simulink model "verify_HeatExchanger_mdl_2019a"  (R2019a)
settings: Solver=ode45  StartTime=0.0  StopTime=5930  MaxStep=1  RelTol=1e-3  EnableMultiTasking=on
libraries: carnot x9
settings Model: Creator=drhf  LastModifiedBy=P41573
settings DataIOCC: SaveFormat=Array  SignalLoggingSaveFormat=ModelDataLogs  SignalLogging=off  DSMLogging=off  ReturnWorkspaceOutputs=off
settings OptimizationCC: ExpressionDepthLimit=2147483647  LifeSpan=inf
settings DebuggingCC: UnderspecifiedInitializationDetection=Classic  MergeDetectMultiDrivingBlocksExec=none  SolverPrmCheckMsg=warning  FcnCallInpInsideContextMsg=warning  StateNameClashWarn=warning  SFUnexpectedBacktrackingDiag=warning  SFNoUnconditionalDefaultTransitionDiag=warning  SFExecutionAtInitializationDiag=none  ArithmeticOperatorsInVariantConditions=warning
settings HardwareCC: ProdBitPerPointer=32  ProdBitPerSizeT=32  ProdBitPerPtrDiffT=32  ProdLargestAtomicFloat=None  ProdIntDivRoundTo=Undefined  ProdEndianess=Unspecified  ProdWordSize=32  ProdHWDeviceType=32-bit Generic
settings ModelReferenceCC: PropagateSignalLabelsOutOfModel=off
settings SFSimCC: SimUseLocalCustomCode=off
settings RTWCC: RTWUseLocalCustomCode=off
settings CodeAppCC: StateflowObjectComments=on
settings GRTTargetCC: TargetLangStandard=C89/C90 (ANSI)  GeneratePreprocessorConditionals=Disable all  CombineOutputUpdateFcns=off  GRTInterface=on
settings ConfigComp: CovMetricSettings=dw  CovHtmlReporting=on  CovSaveCumulativeToWorkspaceVar=on  CovSaveSingleToWorkspaceVar=on  CovExternalEMLEnable=off

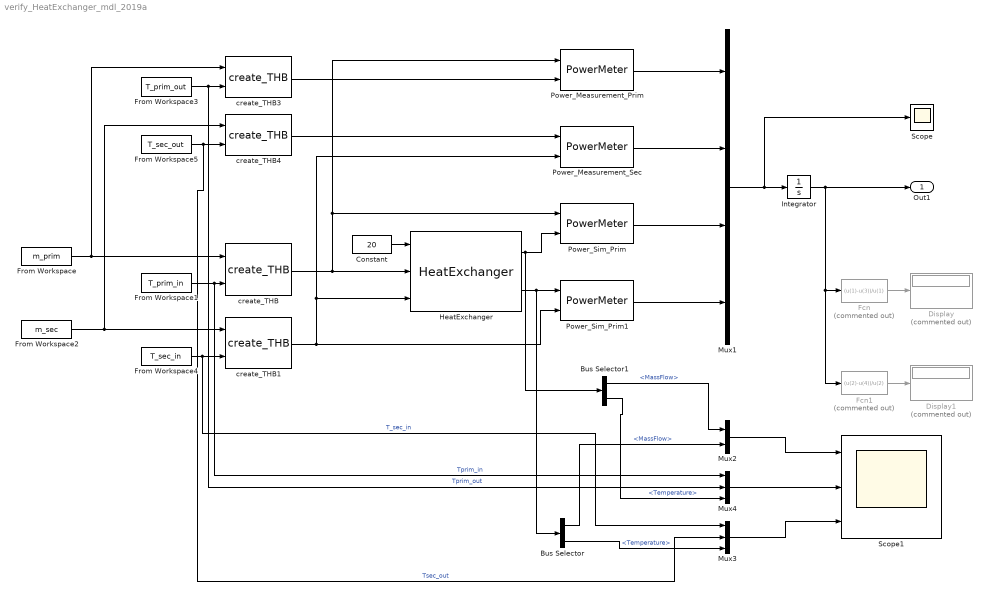
== system verify_HeatExchanger_mdl_2019a ==
  Bus Selector : BusSelector  OutputSignals=MassFlow,Temperature
  Bus Selector1 : BusSelector  OutputSignals=MassFlow,Temperature
  Constant : Constant  Value=20
  Display : Display  Commented=on
  Display1 : Display  Commented=on
  Fcn : Fcn  Commented=on  Expr=(u(1)-u(3))/u(1)
  Fcn1 : Fcn  Commented=on  Expr=(u(2)-u(4))/u(2)
  From Workspace : FromWorkspace  VariableName=m_prim  SampleTime=0
  From Workspace1 : FromWorkspace  VariableName=T_prim_in  SampleTime=0
  From Workspace2 : FromWorkspace  VariableName=m_sec  SampleTime=0
  From Workspace3 : FromWorkspace  VariableName=T_prim_out  SampleTime=0
  From Workspace4 : FromWorkspace  VariableName=T_sec_in  SampleTime=0
  From Workspace5 : FromWorkspace  VariableName=T_sec_out  SampleTime=0
  HeatExchanger : carnot/Source/Heat_Exchanger/HeatExchanger  flowtype=1  ua0=2100  uahot=[0.07 0.41]  uacold=[0.1 0.7]  ualoss=1  cap=8000  linh=20  quah=10  linc=20  quac=10  t0=20
      settings: SourceProductName=Carnot
  Integrator : Integrator
  Mux1 : Mux
  Mux2 : Mux  Inputs=2
  Mux3 : Mux  Inputs=3
  Mux4 : Mux  Inputs=3
  Power_Measurement_Prim : carnot/Control/PowerMeter
      settings: SourceProductName=Carnot
  Power_Measurement_Sec : carnot/Control/PowerMeter
      settings: SourceProductName=Carnot
  Power_Sim_Prim : carnot/Control/PowerMeter
      settings: SourceProductName=Carnot
  Power_Sim_Prim1 : carnot/Control/PowerMeter
      settings: SourceProductName=Carnot
  Scope : Scope
  Scope1 : Scope  NumInputPorts=3
  create_THB{,1,3..4} (4 alike) : carnot/Source/Simple/create_THB  p=1e5  fluid=Water  mix=0  mix2=0  mix3=0  dia=0  hgt=0  mID=No Pressure Drop
      settings: SourceProductName=Carnot
  Out1 : Outport
  wires:
  create_THB/1 -> HeatExchanger/2, Power_Sim_Prim/1, Power_Measurement_Prim/1
  create_THB1/1 -> Power_Measurement_Sec/2, HeatExchanger/3, Power_Sim_Prim1/2
  Constant/1 -> HeatExchanger/1
  From Workspace/1 -> create_THB3/1, create_THB/1
  From Workspace2/1 -> create_THB4/1, create_THB1/1
  From Workspace1/1 -> Mux4/1, create_THB/2  "Tprim_in"
  From Workspace3/1 -> Mux4/2, create_THB3/2  "Tprim_out"
  create_THB3/1 -> Power_Measurement_Prim/2
  Power_Measurement_Prim/1 -> Mux1/1
  Power_Sim_Prim/1 -> Mux1/3
  Power_Measurement_Sec/1 -> Mux1/2
  HeatExchanger/1 -> Bus Selector1/1, Power_Sim_Prim/2
  HeatExchanger/2 -> Bus Selector/1, Power_Sim_Prim1/1
  From Workspace4/1 -> Mux3/1, create_THB1/2  "T_sec_in"
  From Workspace5/1 -> Mux3/2, create_THB4/2  "Tsec_out"
  create_THB4/1 -> Power_Measurement_Sec/1
  Power_Sim_Prim1/1 -> Mux1/4
  Mux1/1 -> Integrator/1, Scope/1
  Integrator/1 -> Out1/1, Fcn1/1, Fcn/1
  Fcn/1 -> Display/1
  Fcn1/1 -> Display1/1
  Bus Selector/1 -> Mux2/2  "<MassFlow>"
  Bus Selector/2 -> Mux3/3  "<Temperature>"
  Bus Selector1/1 -> Mux2/1  "<MassFlow>"
  Bus Selector1/2 -> Mux4/3  "<Temperature>"
  Mux2/1 -> Scope1/1
  Mux3/1 -> Scope1/3
  Mux4/1 -> Scope1/2
